simulink model "Tones_1"  (R2022a)
settings: Solver=FixedStepAuto  StartTime=0.0  StopTime=inf  FixedStep=TSI  RelTol=1e-3  EnableMultiTasking=on
InitFcn:
  | Ts = 1/5000
undefined symbols (not defined in the file): TSI
libraries: arduinolib x1
settings Model: ExtModeTrigDuration=2  Creator=mshafiqu  LastModifiedBy=Kostas Tsakalis
settings SolverCC: AlgebraicLoopSolver=TrustRegion
settings DataIOCC: LimitDataPoints=on  ReturnWorkspaceOutputs=off
settings OptimizationCC: LifeSpan=1  MaxStackSize=64  EfficientTunableParamExpr=on
settings DebuggingCC: UnconnectedInputMsg=warning  UnconnectedOutputMsg=warning  UnconnectedLineMsg=warning  AllowSymbolicDim=off  SFUnexpectedBacktrackingDiag=warning  SFNoUnconditionalDefaultTransitionDiag=warning  SFExecutionAtInitializationDiag=none  SFMachineParentedDataDiag=warning  ArithmeticOperatorsInVariantConditions=warning
settings HardwareCC: ProdBitPerPointer=32  ProdBitPerSizeT=32  ProdBitPerPtrDiffT=32  ProdLargestAtomicInteger=Long  ProdLargestAtomicFloat=Double  ProdWordSize=32  ProdHWDeviceType=ARM Compatible->ARM Cortex  UseEmbeddedCoderFeatures=off  UseSimulinkCoderFeatures=off
settings ModelReferenceCC: PropagateSignalLabelsOutOfModel=off
settings SFSimCC: SimUseLocalCustomCode=off  MATLABDynamicMemAlloc=off  CustomCodeUndefinedFunction=UseInterfaceOnly
settings RTWCC: SystemTargetFile=ert.tlc  HardwareBoard=Arduino Due  TemplateMakefile=ert_default_tmf  RTWUseLocalCustomCode=off  Toolchain=Arduino ARM  BuildConfiguration=Faster Runs
settings CodeAppCC: IgnoreCustomStorageClasses=off  StateflowObjectComments=on
settings ERTTargetCC: MultiwordLength=2048  SupportContinuousTime=on  SupportNonInlinedSFcns=on  SupportVariableSizeSignals=on  ConvertIfToSwitch=off  SuppressUnreachableDefaultCases=off
settings ConfigComp: CovMetricSettings=dw  CovSaveCumulativeToWorkspaceVar=on  CovSaveSingleToWorkspaceVar=on  CovExternalEMLEnable=off

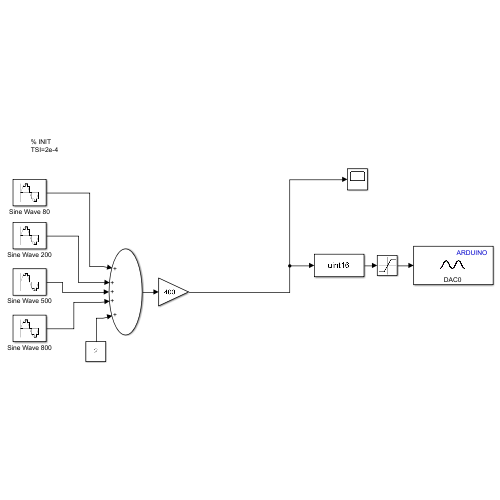
[thumbnail: Simulink's stored preview of the top-level diagram]
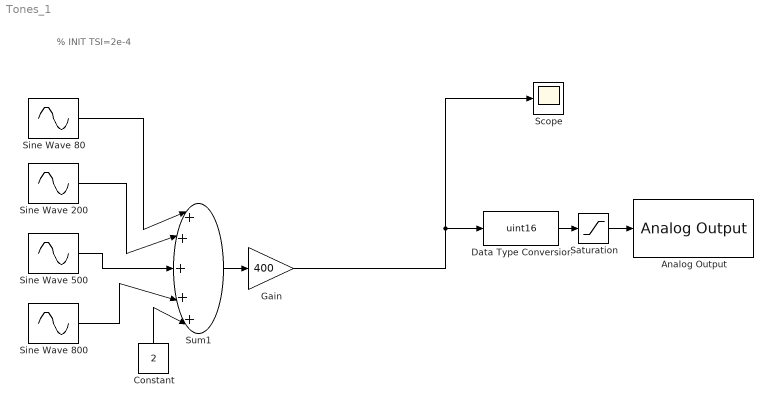
== system Tones_1 ==
  note: % INIT
      | TSI=2e-4
  Analog Output : arduinolib/Analog Output  DACpin=DAC0  blockPlatform=arduino
      settings: SourceProductBaseCode=ARDUINO
  Constant : Constant  Value=2  SampleTime=Ts
  Data Type Conversion : DataTypeConversion  OutDataTypeStr=uint16  SaturateOnIntegerOverflow=off  RndMeth=Floor
  Gain : Gain  Gain=400
  Saturation : Saturate  UpperLimit=4095  LowerLimit=0
  Scope : Scope
  Sine Wave 200 : Sin  Amplitude=0.5  Frequency=2*pi*200  Samples=125  SampleTime=TSI
  Sine Wave 500 : Sin  Amplitude=0.5  Frequency=2*pi*500  Samples=125  SampleTime=TSI
  Sine Wave 80 : Sin  Amplitude=0.5  Frequency=2*pi*80  Samples=125  SampleTime=TSI
  Sine Wave 800 : Sin  Amplitude=0.5  Frequency=2*pi*800  Samples=125  SampleTime=TSI
  Sum1 : Sum  Inputs=|+++++|
  wires:
  Data Type Conversion/1 -> Saturation/1
  Sine Wave 80/1 -> Sum1/1
  Gain/1 -> Scope/1, Data Type Conversion/1
  Sum1/1 -> Gain/1
  Sine Wave 200/1 -> Sum1/2
  Constant/1 -> Sum1/5
  Sine Wave 500/1 -> Sum1/3
  Sine Wave 800/1 -> Sum1/4
  Saturation/1 -> Analog Output/1
